simulink model "armDynamicsV2_WTZMIC001"  (R2021a)
settings: Solver=ode4  StartTime=0.0  StopTime=5  FixedStep=0.01  MaxStep=0.01  RelTol=1e-3
settings Model: Creator=kukho  LastModifiedBy=michk
settings SolverCC: AutoInsertRateTranBlk=on

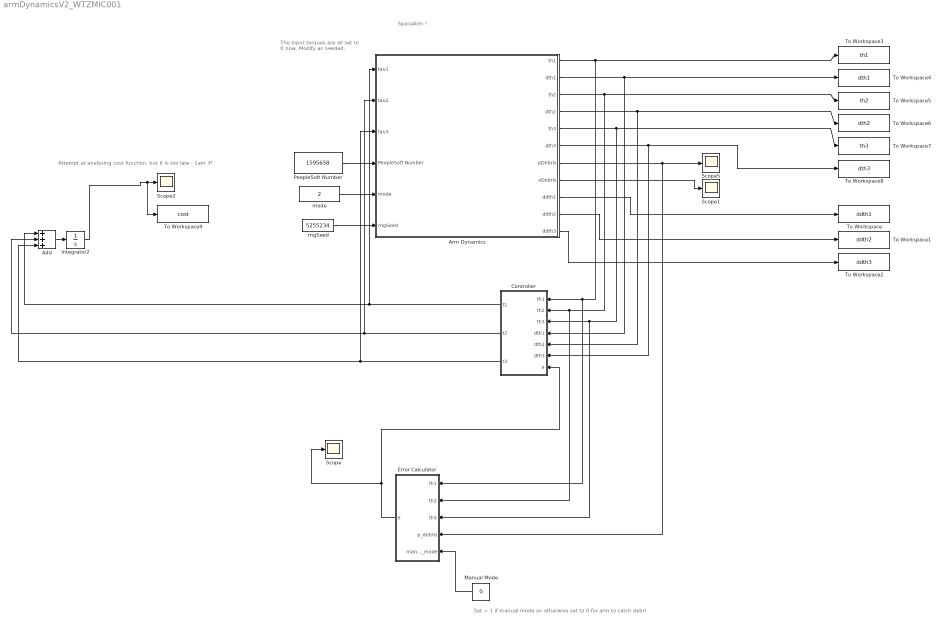
== system armDynamicsV2_WTZMIC001 ==
  note: Attempt at analysing cost function. but it is too late - 1am :P
  note: Set = 1 if manual mode on otherwise set to 0 for arm to catch debri
  note: SpaceArm !
  note: The input torques are all set to 0 now. Modify as needed.
  Add : Sum  Inputs=+++
  Arm Dynamics : Subsystem
      mask Display: image('C:\Users\kukho\Desktop\2021\Teaching Assistant\Project\Project Final\Images\modelimage.png'); % Use "Edit Image" on toolstrip to change.
  Controller : MATLAB Function  TreatAsAtomicUnit=on
  Error Calculator : MATLAB Function  TreatAsAtomicUnit=on
  Integrator2 : Integrator
  Manual Mode : Constant  Value=0
  PeopleSoft Number : Constant  Value=1595658
  Scope{,1..2,5} (4 alike) : Scope
  To Workspace : ToWorkspace  VariableName=ddth1  SampleTime=-1
  To Workspace1 : ToWorkspace  VariableName=ddth2  SampleTime=-1
  To Workspace2 : ToWorkspace  VariableName=ddth3  SampleTime=-1
  To Workspace3 : ToWorkspace  VariableName=th1  SampleTime=-1
  To Workspace4 : ToWorkspace  VariableName=dth1  SampleTime=-1
  To Workspace5 : ToWorkspace  VariableName=th2  SampleTime=-1
  To Workspace6 : ToWorkspace  VariableName=dth2  SampleTime=-1
  To Workspace7 : ToWorkspace  VariableName=th3  SampleTime=-1
  To Workspace8 : ToWorkspace  VariableName=dth3  SampleTime=-1
  To Workspace9 : ToWorkspace  VariableName=cost  SampleTime=-1
  mode : Constant  Value=2
  rngSeed : Constant  Value=5255234
  wires:
  Controller/1(t1) -> Add/1, Arm Dynamics/1(tau1)
  Controller/2(t2) -> Add/2, Arm Dynamics/2(tau2)
  Controller/3(t3) -> Add/3, Arm Dynamics/3(tau3)
  PeopleSoft Number/1 -> Arm Dynamics/4(PeopleSoft Number)
  mode/1 -> Arm Dynamics/5(mode)
  rngSeed/1 -> Arm Dynamics/6(rngSeed)
  Arm Dynamics/7(pDebris) -> Error Calculator/4(p_debris), Scope5/1
  Arm Dynamics/8(vDebris) -> Scope1/1
  Arm Dynamics/5(th3) -> Error Calculator/3(th3), Controller/3(th3), To Workspace7/1
  Arm Dynamics/1(th1) -> Controller/1(th1), Error Calculator/1(th1), To Workspace3/1
  Arm Dynamics/4(dth2) -> Controller/5(dth2), To Workspace6/1
  Arm Dynamics/6(dth3) -> Controller/6(dth3), To Workspace8/1
  Arm Dynamics/2(dth1) -> Controller/4(dth1), To Workspace4/1
  Arm Dynamics/3(th2) -> Error Calculator/2(th2), Controller/2(th2), To Workspace5/1
  Arm Dynamics/9(ddth1) -> To Workspace/1
  Arm Dynamics/10(ddth2) -> To Workspace1/1
  Arm Dynamics/11(ddth3) -> To Workspace2/1
  Error Calculator/1(e) -> Controller/7(e), Scope/1
  Integrator2/1 -> To Workspace9/1, Scope2/1
  Add/1 -> Integrator2/1
  Manual Mode/1 -> Error Calculator/5(manual_mode)

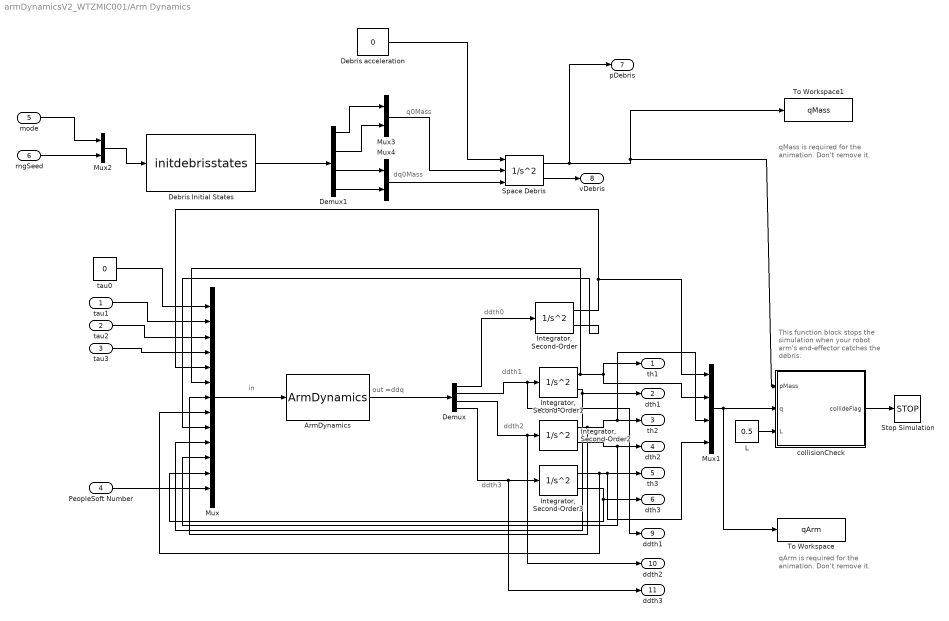
== system armDynamicsV2_WTZMIC001/Arm Dynamics ==
  note: dq0Mass
  note: q0Mass
  note: in
  note: out =ddq
  note: ddth3
  note: ddth2
  note: ddth1
  note: ddth0
  note: This function block stops the simulation when your robot arm's end-effector catches the debris.
  note: qMass is required for the animation. Don't remove it.
  note: qArm is required for the animation. Don't remove it.
  tau1 : Inport
  tau2 : Inport  Port=2
  tau3 : Inport  Port=3
  PeopleSoft Number : Inport  Port=4
  mode : Inport  Port=5
  rngSeed : Inport  Port=6
  ArmDynamics : MATLABFcn  MATLABFcn=ArmDynamics  OutputDimensions=4
  Debris Initial States : MATLABFcn  MATLABFcn=initdebrisstates  OutputDimensions=4
  Debris acceleration : Constant  Value=0
  Demux : Demux
  Demux1 : Demux
  "Integrator, Second-Order" : SecondOrderIntegrator
  "Integrator, Second-Order1" : SecondOrderIntegrator  ICX=-1*pi/2
  "Integrator, Second-Order2" : SecondOrderIntegrator
  "Integrator, Second-Order3" : SecondOrderIntegrator
  L : Constant  Value=0.5
  Mux : Mux  Inputs=13
  Mux1 : Mux
  Mux2 : Mux  Inputs=2
  Mux3 : Mux  Inputs=2
  Mux4 : Mux  Inputs=2
  Space Debris : SecondOrderIntegrator  ICSourceX=external  ICX=q0Mass  ICSourceDXDT=external  ICDXDT=dq0Mass
  Stop Simulation : Stop
  To Workspace : ToWorkspace  VariableName=qArm  SaveFormat=Structure With Time  SampleTime=0.01
  To Workspace1 : ToWorkspace  VariableName=qMass  SaveFormat=Structure With Time  SampleTime=0.01
  collisionCheck : MATLAB Function  TreatAsAtomicUnit=on
  tau0 : Constant  Value=0
  th1 : Outport
  dth1 : Outport  Port=2
  th2 : Outport  Port=3
  dth2 : Outport  Port=4
  th3 : Outport  Port=5
  dth3 : Outport  Port=6
  pDebris : Outport  Port=7
  vDebris : Outport  Port=8
  ddth1 : Outport  Port=9
  ddth2 : Outport  Port=10
  ddth3 : Outport  Port=11
  wires:
  "Integrator, Second-Order1"/2 -> dth1/1, Mux/10
  "Integrator, Second-Order1"/1 -> Mux/6, th1/1, Mux1/2
  "Integrator, Second-Order3"/2 -> dth3/1, Mux/12
  Demux/4 -> ddth3/1, "Integrator, Second-Order3"/1
  "Integrator, Second-Order"/1 -> Mux/5, Mux1/1
  Mux1/1 -> To Workspace/1, collisionCheck/2(q)
  "Integrator, Second-Order2"/1 -> Mux/7, th2/1, Mux1/3
  Mux3/1 -> Space Debris/2
  Space Debris/2 -> vDebris/1
  Demux/2 -> ddth1/1, "Integrator, Second-Order1"/1
  Demux/3 -> ddth2/1, "Integrator, Second-Order2"/1
  "Integrator, Second-Order"/2 -> Mux/9
  Demux1/3 -> Mux4/1
  tau3/1 -> Mux/4
  tau2/1 -> Mux/3
  "Integrator, Second-Order2"/2 -> dth2/1, Mux/11
  Mux4/1 -> Space Debris/3
  Demux1/4 -> Mux4/2
  Demux1/1 -> Mux3/1
  Space Debris/1 -> pDebris/1, To Workspace1/1, collisionCheck/1(pMass)
  Mux2/1 -> Debris Initial States/1
  PeopleSoft Number/1 -> Mux/13
  rngSeed/1 -> Mux2/2
  mode/1 -> Mux2/1
  Debris acceleration/1 -> Space Debris/1
  "Integrator, Second-Order3"/1 -> Mux/8, th3/1, Mux1/4
  ArmDynamics/1 -> Demux/1
  Demux/1 -> "Integrator, Second-Order"/1
  Mux/1 -> ArmDynamics/1
  collisionCheck/1(collideFlag) -> Stop Simulation/1
  tau1/1 -> Mux/2
  Demux1/2 -> Mux3/2
  tau0/1 -> Mux/1
  L/1 -> collisionCheck/3(L)
  Debris Initial States/1 -> Demux1/1

== matlab function armDynamicsV2_WTZMIC001/Controller ==
  data: th1 input; t1 output; th2 input; th3 input; dth1 input; dth2 input; dth3 input; t2 output; t3 output; e input
function [t1,t2,t3]= fcn(th1, th2, th3, dth1, dth2, dth3, e)

m = 1;
I = 0.1;  
L = 0.5;
Kp = 65     %gains
Kd = 13
e1 = e(1)   
e2 = e(2)
e3 = e(3)
de1 = -dth1  %this is the parameters i used for the derivative of the error instead of a block or extra formula
de2 = -dth2
de3 = -dth3

%to find these tau equations I found them in the Sys_dynamics script
%symbolically. Here I sub in the values to them and actually work them out.

t1 = (43179*dth1)/10000 + (Kd*de2 + Kp*e2)*(2*I + (3*L^2*m)/2 + (L^2*m*cos(th2 + th3))/2 + (3*L^2*m*cos(th2))/2 + L^2*m*cos(th3)) + (Kd*de1 + Kp*e1)*(3*I + (15*L^2*m)/4 + L^2*m*cos(th2 + th3) + 3*L^2*m*cos(th2) + L^2*m*cos(th3)) - dth3*(dth3*((L^2*m*sin(th2 + th3))/2 + (L^2*m*sin(th3))/2) + (L^2*dth2*m*sin(th2 + th3))/2) + (Kd*de3 + Kp*e3)*(I + (L^2*m)/4 + (L^2*m*cos(th2 + th3))/2 + (L^2*m*cos(th3))/2) - dth1*(dth3*(L^2*m*sin(th2 + th3) + L^2*m*sin(th3)) + dth2*(L^2*m*sin(th2 + th3) + 3*L^2*m*sin(th2))) - dth2*(dth3*((L^2*m*sin(th2 + th3))/2 + L^2*m*sin(th3)) + dth2*((L^2*m*sin(th2 + th3))/2 + (3*L^2*m*sin(th2))/2))
t2 = (43179*dth2)/10000 + (Kd*de1 + Kp*e1)*(2*I + (3*L^2*m)/2 + (L^2*m*cos(th2 + th3))/2 + (3*L^2*m*cos(th2))/2 + L^2*m*cos(th3)) + (Kd*de3 + Kp*e3)*(I + (L^2*m)/4 + (L^2*m*cos(th3))/2) + (Kd*de2 + Kp*e2)*(2*I + (3*L^2*m)/2 + L^2*m*cos(th3)) - (L^2*m*(dth3^2*sin(th3) - 3*dth1^2*sin(th2) - dth1^2*sin(th2 + th3) + 2*dth1*dth3*sin(th3) + 2*dth2*dth3*sin(th3)))/2
t3 = (43179*dth3)/10000 + (Kd*de2 + Kp*e2)*(I + (L^2*m)/4 + (L^2*m*cos(th3))/2) + (Kd*de1 + Kp*e1)*(I + (L^2*m)/4 + (L^2*m*cos(th2 + th3))/2 + (L^2*m*cos(th3))/2) + ((m*L^2)/4 + I)*(Kd*de3 + Kp*e3) + (L^2*m*(dth1^2*sin(th3) + dth2^2*sin(th3) + dth1^2*sin(th2 + th3) + 2*dth1*dth2*sin(th3)))/2

== matlab function armDynamicsV2_WTZMIC001/Arm Dynamics/collisionCheck ==
  data: pMass input; collideFlag output; q input; L input
function collideFlag = fcn(pMass, q, L)
thresh = 0.1;   %threshold for vacuum to suck up debris

th0 = q(1);
th1 = q(2);
th2 = q(3);
th3 = q(4);

pEnd = [L*(cos(th0 + th1 + th2) + cos(th0 + th1 + th2 + th3) + cos(th0 + th1));...
        L*(sin(th0 + th1 + th2) + sin(th0 + th1 + th2 + th3) + sin(th0 + th1))];


% Calculate Euclidean Distance
dist = pMass-pEnd;

if norm(dist) <= thresh
    
    collideFlag = 1;
else
    collideFlag = 0;
end

== matlab function armDynamicsV2_WTZMIC001/Error Calculator ==
  data: th1 input; th2 input; e output; th3 input; p_debris input; manual_mode input
function e = fcn(th1, th2, th3, p_debris, manual_mode)
L = 0.5

debris_x = p_debris(1)
debris_y = p_debris(2)

% setpoint in this case is an angle
setpoint = atan(debris_y/debris_x)
% If debris approaches from left isde the angle should be adjusted
if debris_x < 0
    setpoint = -pi + atan(debris_y/debris_x)
end
if manual_mode == 1        %Mode where link should go upright
    setpoint = pi/2
end
e = [setpoint - th1;-th2;-th3]
